simulink model "Scatola3"  (R2019a)
settings: Solver=VariableStepAuto  StartTime=0.0  StopTime=10.0  RelTol=1e-3
settings Model: Creator=anton  LastModifiedBy=anton

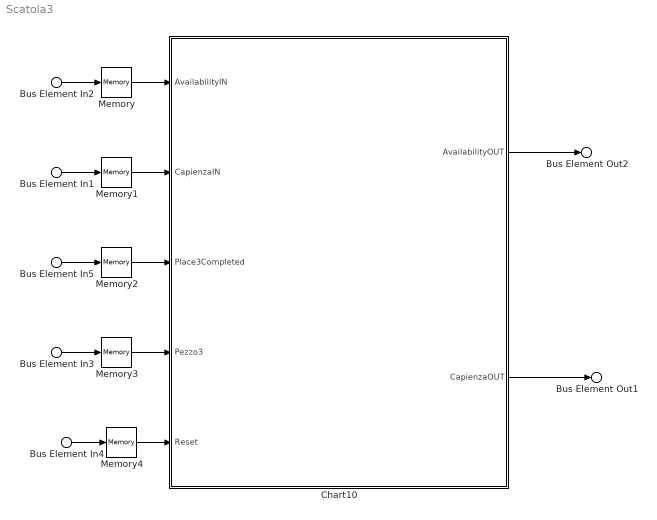
== system Scatola3 ==
  Bus Element In1 : Inport  PortName=CapienzaIN
  Bus Element In2 : Inport  Port=2  PortName=AvailabilityIN
  Bus Element In4 : Inport  Port=3  PortName=Reset
  Bus Element In5 : Inport  Port=4  PortName=Place3Completed
  Bus Element In3 : Inport  Port=5  PortName=Pezzo3
  Chart10 : Stateflow chart  BlockKeywords=__PRM__SERIALIZED__DATA__:Stateflow Chart,Stateflow Diagram  TreatAsAtomicUnit=on
  Memory{,1..4} (5 alike) : Memory
  Bus Element Out1 : Outport  PortName=Capienza3OUT
  Bus Element Out2 : Outport  Port=2  PortName=AvailabilityOUT
  wires:
  Chart10/1(AvailabilityOUT) -> Bus Element Out2/1
  Chart10/2(CapienzaOUT) -> Bus Element Out1/1
  Bus Element In2/1 -> Memory/1
  Memory/1 -> Chart10/1(AvailabilityIN)
  Bus Element In1/1 -> Memory1/1
  Memory1/1 -> Chart10/2(CapienzaIN)
  Bus Element In5/1 -> Memory2/1
  Memory2/1 -> Chart10/3(Place3Completed)
  Bus Element In3/1 -> Memory3/1
  Memory3/1 -> Chart10/4(Pezzo3)
  Bus Element In4/1 -> Memory4/1
  Memory4/1 -> Chart10/5(Reset)

== stateflow chart Scatola3/Chart10 ==
  state Idle
    CapienzaOUT=0;
    AvailabilityOUT=AvailabilityIN;
    pause(0.1);
  state Capienza6
    CapienzaOUT=0;
    AvailabilityOUT=AvailabilityIN;
    pause(0.1);
  state Waiting5
  state Capienza5
    CapienzaOUT=1;
    AvailabilityOUT=AvailabilityIN;
    pause(0.1);
  state Waiting4
  state Capienza4
    CapienzaOUT=2;
    AvailabilityOUT=AvailabilityIN;
    pause(0.1);
  state Waiting3
  state Capienza3
    CapienzaOUT=3;
    AvailabilityOUT=AvailabilityIN;
    pause(0.1);
  state Waiting2
  state Capienza2
    CapienzaOUT=4;
    AvailabilityOUT=AvailabilityIN;
    pause(0.1);
  state Waiting
  state Capienza1
    CapienzaOUT=5;
    AvailabilityOUT=AvailabilityIN;
    pause(0.1);
  state Waiting1
  state Capienza0
    CapienzaOUT=6;
    AvailabilityOUT=AvailabilityIN;
    pause(0.1);
  (default) -> Idle
  Capienza0 -> Idle : [CapienzaIN==1]
  Idle -> Capienza6
  Capienza6 -> Waiting5 : [Place3Completed==1]
  Waiting5 -> Capienza5 : [Reset==1]
  Capienza5 -> Waiting4 : [Place3Completed==1]
  Waiting4 -> Capienza4 : [Reset==1]
  Capienza4 -> Waiting3 : [Place3Completed==1]
  Waiting3 -> Capienza3 : [Reset==1]
  Capienza3 -> Waiting2 : [Place3Completed==1]
  Waiting2 -> Capienza2 : [Reset==1]
  Capienza2 -> Waiting : [Place3Completed==1]
  Waiting -> Capienza1 : [Reset==1]
  Capienza1 -> Waiting1 : [Place3Completed==1]
  Waiting1 -> Capienza0 : [Reset==1]
  data: AvailabilityIN input; CapienzaIN input; Place3Completed input; Pezzo3 input; Reset input; AvailabilityOUT output; CapienzaOUT output
